simulink model "DHthuan"  (R2020a)
settings: Solver=VariableStepAuto  StartTime=0.0  StopTime=10.0  RelTol=1e-3
settings Model: Creator=dell  LastModifiedBy=dell

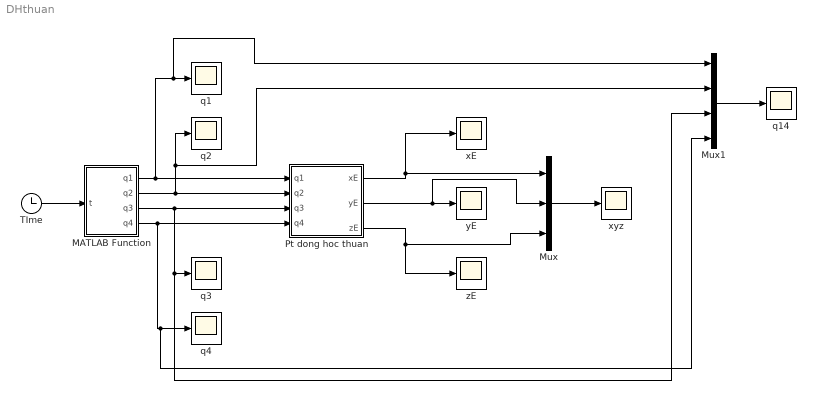
== system DHthuan ==
  MATLAB Function : MATLAB Function  TreatAsAtomicUnit=on
  Mux : Mux  Inputs=3
  Mux1 : Mux
  "Pt dong hoc thuan " : MATLAB Function  TreatAsAtomicUnit=on
  TIme : Clock
  q{1..4,14} (5 alike) : Scope
  xE : Scope
  xyz : Scope
  yE : Scope
  zE : Scope
  wires:
  "Pt dong hoc thuan "/2(yE) -> Mux/2, yE/1
  "Pt dong hoc thuan "/3(zE) -> Mux/3, zE/1
  MATLAB Function/3(q3) -> Mux1/3, q3/1, "Pt dong hoc thuan "/3(q3)
  MATLAB Function/2(q2) -> Mux1/2, q2/1, "Pt dong hoc thuan "/2(q2)
  MATLAB Function/1(q1) -> Mux1/1, q1/1, "Pt dong hoc thuan "/1(q1)
  TIme/1 -> MATLAB Function/1(t)
  MATLAB Function/4(q4) -> Mux1/4, q4/1, "Pt dong hoc thuan "/4(q4)
  "Pt dong hoc thuan "/1(xE) -> Mux/1, xE/1
  Mux/1 -> xyz/1
  Mux1/1 -> q14/1

== matlab function DHthuan/MATLAB Function ==
  data: t input; q1 output; q2 output; q3 output; q4 output
function [q1,q2,q3,q4] = fcn(t)
q1= sin(t);
q2=(pi/2)*sin(t);
q3=(pi/3)*cos(t);
q4= (pi/6)*sin(t/4);
end

== matlab function DHthuan/Pt dong hoc thuan  ==
  data: q1 input; xE output; q2 input; q3 input; q4 input; yE output; zE output
function [xE,yE,zE] = fcn(q1,q2,q3,q4)
L1 = 0.1;
L2 = 0.4;
L3 = 0.3;
L4 = 0.3;
xE = 0;
yE = (-sin(q2) * cos(q3) - cos(q2) * sin(q3)) * L4 * cos(q4) + (sin(q2) * sin(q3) - cos(q2) * cos(q3)) * L4 * sin(q4) - sin(q2) * L3 * cos(q3) - cos(q2) * L3 * sin(q3) - L2 * sin(q2);
zE = (cos(q2) * cos(q3) - sin(q2) * sin(q3)) * L4 * cos(q4) + (-sin(q2) * cos(q3) - cos(q2) * sin(q3)) * L4 * sin(q4) + cos(q2) * L3 * cos(q3) - sin(q2) * L3 * sin(q3) + L2 * cos(q2) + L1 + q1;
end
